simulink model "P_Respuesta_Ideal_2P"  (R2021b)
settings: Solver=VariableStepAuto  StartTime=0.0  StopTime=50  RelTol=1e-3
libraries: cstblocks x4
settings Model: Creator=parra  LastModifiedBy=parra

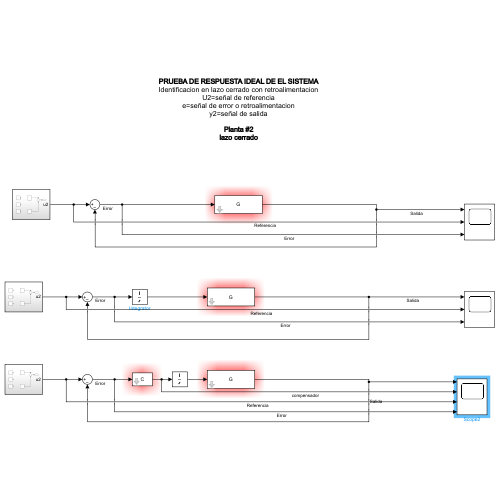
[thumbnail: Simulink's stored preview of the top-level diagram]
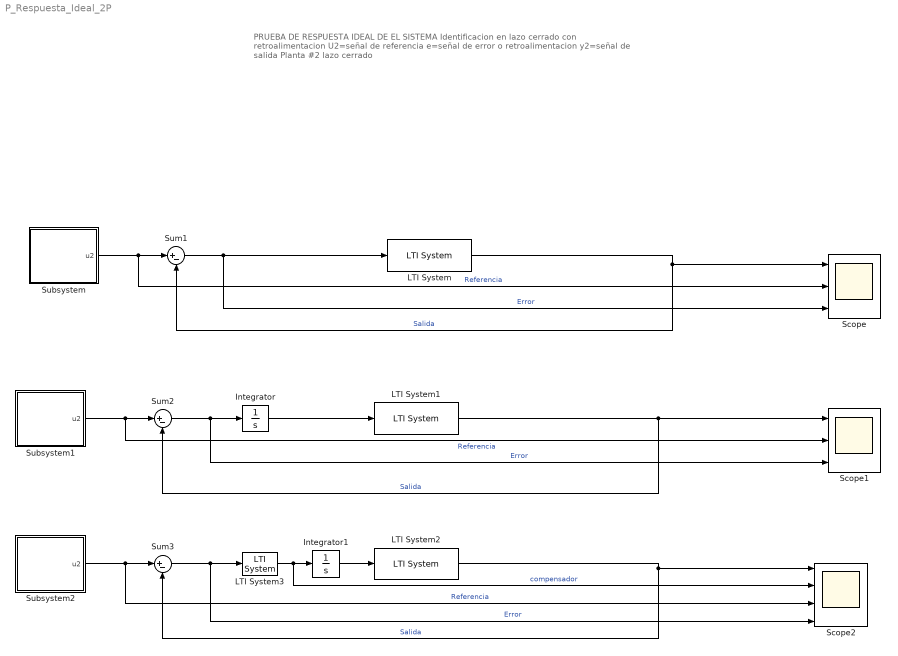
== system P_Respuesta_Ideal_2P ==
  note: PRUEBA DE RESPUESTA IDEAL DE EL SISTEMA
      | Identificacion en lazo cerrado con retroalimentacion
      | U2=señal de referencia
      | e=señal de error o retroalimentacion
      | y2=señal de salida
      |
      | Planta #2
      | lazo cerrado
  Integrator : Integrator
  Integrator1 : Integrator
  LTI System : cstblocks/LTI System  sys=G  IC=[]
  LTI System1 : cstblocks/LTI System  sys=G  IC=[]
  LTI System2 : cstblocks/LTI System  sys=G  IC=[]
  LTI System3 : cstblocks/LTI System  sys=C  IC=[]
  Scope : Scope  NumInputPorts=3
  Scope1 : Scope  NumInputPorts=3
  Scope2 : Scope  NumInputPorts=4
  Subsystem : Subsystem
  Subsystem1 : Subsystem
  Subsystem2 : Subsystem
  Sum1 : Sum  Inputs=|+-
  Sum2 : Sum  Inputs=|+-
  Sum3 : Sum  Inputs=|+-
  wires:
  Subsystem/1(u2) -> Scope/2, Sum1/1  "Referencia"
  Sum1/1 -> LTI System/1, Scope/3  "Error"
  LTI System/1 -> Sum1/2, Scope/1  "Salida"
  Subsystem1/1(u2) -> Scope1/2, Sum2/1  "Referencia"
  Sum2/1 -> Integrator/1, Scope1/3  "Error"
  LTI System1/1 -> Sum2/2, Scope1/1  "Salida"
  Integrator/1 -> LTI System1/1
  Integrator1/1 -> LTI System2/1
  Subsystem2/1(u2) -> Scope2/3, Sum3/1  "Referencia"
  LTI System2/1 -> Sum3/2, Scope2/1  "Salida"
  Sum3/1 -> Scope2/4, LTI System3/1  "Error"
  LTI System3/1 -> Scope2/2, Integrator1/1  "compensador"

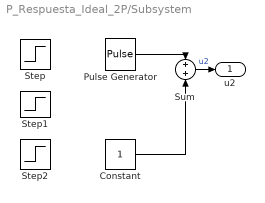
== system P_Respuesta_Ideal_2P/Subsystem ==
  Constant : Constant
  Pulse Generator : DiscretePulseGenerator  Amplitude=0.5  Period=2500  PulseWidth=1250  SampleTime=0.01
  Step : Step  Time=10  Before=0.5  SampleTime=0.01
  Step1 : Step  Time=13  Before=1  After=1.5  SampleTime=0.01
  Step2 : Step  Time=16  Before=1  After=1.5  SampleTime=0.01
  Sum : Sum
  u2 : Outport
  wires:
  Sum/1 -> u2/1  "u2"
  Pulse Generator/1 -> Sum/1
  Constant/1 -> Sum/2

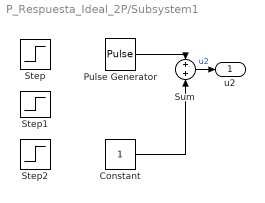
== system P_Respuesta_Ideal_2P/Subsystem1 ==
  Constant : Constant
  Pulse Generator : DiscretePulseGenerator  Amplitude=0.5  Period=2500  PulseWidth=1250  SampleTime=0.01
  Step : Step  Time=10  Before=0.5  SampleTime=0.01
  Step1 : Step  Time=13  Before=1  After=1.5  SampleTime=0.01
  Step2 : Step  Time=16  Before=1  After=1.5  SampleTime=0.01
  Sum : Sum
  u2 : Outport
  wires:
  Sum/1 -> u2/1  "u2"
  Pulse Generator/1 -> Sum/1
  Constant/1 -> Sum/2

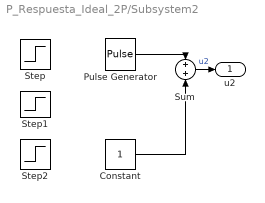
== system P_Respuesta_Ideal_2P/Subsystem2 ==
  Constant : Constant
  Pulse Generator : DiscretePulseGenerator  Amplitude=0.5  Period=2500  PulseWidth=1250  SampleTime=0.01
  Step : Step  Time=10  Before=0.5  SampleTime=0.01
  Step1 : Step  Time=13  Before=1  After=1.5  SampleTime=0.01
  Step2 : Step  Time=16  Before=1  After=1.5  SampleTime=0.01
  Sum : Sum
  u2 : Outport
  wires:
  Sum/1 -> u2/1  "u2"
  Pulse Generator/1 -> Sum/1
  Constant/1 -> Sum/2
